simulink model "platforma3"  (Simulink 7.9)
settings: Solver=ode23  StartTime=0.0  StopTime=60  RelTol=1e-8
values from neighbouring files (symbols this model uses):
  a = 0.365    [REX.m]
  b = 0.365    [REX.m]
  c = 0.387    [REX.m]
  d = 0.387    [REX.m]
  enk = 0    [REX.m]
  eta_G = 0.72    [przekladnia_203126.m]    (also in przekladnia_203128.m = 0.64; przekladnia_223095.m = 0.75)
  fr = 0.1    [REX.m]
  g = 9.81    [REX.m]
  i = 113    [przekladnia_203126.m]    (also in przekladnia_203128.m = 150; przekladnia_223095.m)
  I_0 = 0.834    [silnik_136211.m]    (also in silnik_305014.m = 0.485)
  Ik = 0.15    [REX.m]
  Ip = I    (= 4.4)    [REX.m]
  J_R = 209*10^(-3)*(10^(-2))^2    (= 2.09e-05)    [silnik_136211.m]    (also in silnik_305014.m = 3.3e-06)
  JC = 0.15*10^-3    (= 0.00015)    [przekladnia_203126.m]    (also in przekladnia_203128.m; przekladnia_223095.m)
  k1 = 1    [REX.m]
  k2 = 1    [REX.m]
  k_M = 32.8 *10^(-3)    (= 0.0328)    [silnik_136211.m]    (also in silnik_305014.m = 0.0205)
  Kd = 300    [REX.m]
  mi = 0.9    [REX.m]
  mp = 45    [REX.m]
  n_0 = 9730    [silnik_136211.m]    (also in silnik_305014.m = 16700)
  n_n = 10400    [silnik_136211.m]    (also in silnik_305014.m = 16200)
  omega = 0.15    [REX.m]
  R = 10    [REX.m]
  r = 0.127    [REX.m]
  tt = 0.387    [REX.m]
  vd = 1.5    [REX.m]
undefined symbols (not defined in the file or in its folder): dm, F, f0, f1, Irstop, sigB, sigG, sigR, v0
settings Model: Creator=mat  LastModifiedBy=student
settings DebuggingCC: FcnCallInpInsideContextMsg=Use local settings
settings GRTTargetCC: CombineOutputUpdateFcns=off  GRTInterface=on

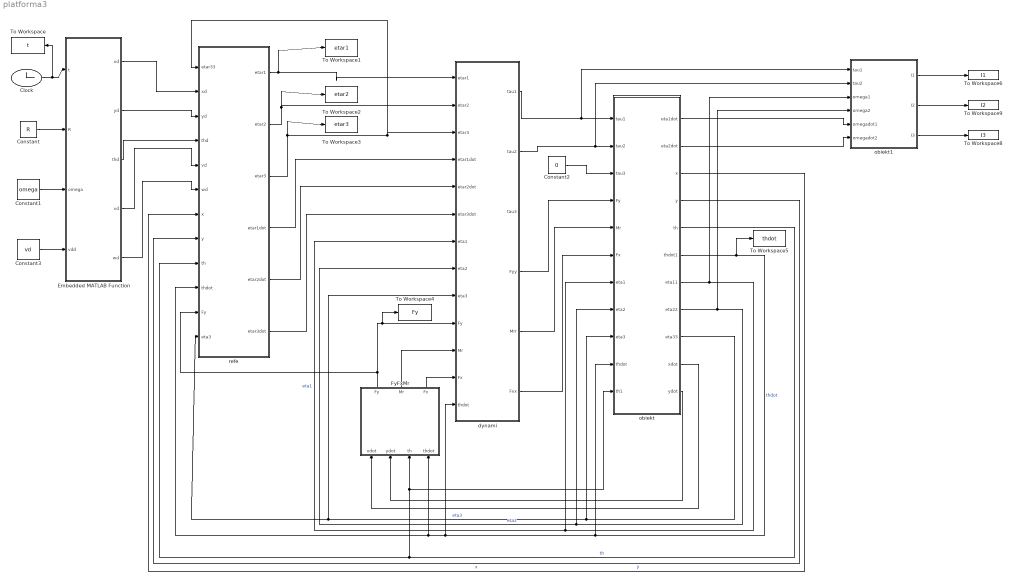
== system platforma3 ==
  Clock : Clock
  Constant : Constant  Value=R
  Constant1 : Constant  Value=omega
  Constant2 : Constant  Value=0
  Constant3 : Constant  Value=vd
  Embedded MATLAB Function : MATLAB Function  TreatAsAtomicUnit=on
  FyFxMr : Subsystem
  To Workspace : ToWorkspace  VariableName=t  SampleTime=-1
  To Workspace1 : ToWorkspace  VariableName=etar1  SampleTime=-1
  To Workspace2 : ToWorkspace  VariableName=etar2  SampleTime=-1
  To Workspace3 : ToWorkspace  VariableName=etar3  SampleTime=-1
  To Workspace4 : ToWorkspace  VariableName=Fy  SampleTime=-1
  To Workspace5 : ToWorkspace  VariableName=thdot  SampleTime=-1
  To Workspace6 : ToWorkspace  VariableName=I1  SampleTime=-1
  To Workspace8 : ToWorkspace  VariableName=I3  SampleTime=-1
  To Workspace9 : ToWorkspace  VariableName=I2  SampleTime=-1
  dynami : Subsystem
  obiekt : Subsystem
  obiekt1 : Subsystem
  refe : Subsystem
  wires:
  Clock/1 -> Embedded MATLAB Function/1(t), To Workspace/1
  Constant/1 -> Embedded MATLAB Function/2(R)
  Constant1/1 -> Embedded MATLAB Function/3(omega)
  dynami/1(tau1) -> obiekt/1(tau1), obiekt1/1(tau1)
  dynami/2(tau2) -> obiekt/2(tau2), obiekt1/2(tau2)
  FyFxMr/3(Fx) -> dynami/12(Fx)
  dynami/4(Fyy) -> obiekt/4(Fy)
  dynami/5(Mrr) -> obiekt/5(Mr)
  dynami/6(Fxx) -> obiekt/6(Fx)
  obiekt/9(eta33) -> obiekt/9(eta3), dynami/9(eta3), refe/12(eta3)  "eta3"
  obiekt/8(eta22) -> obiekt1/4(omega2), obiekt/8(eta2), dynami/8(eta2)  "eta2"
  obiekt/7(eta11) -> obiekt1/3(omega1), obiekt/7(eta1), dynami/7(eta1)  "eta1"
  Embedded MATLAB Function/1(xd) -> refe/2(xd)
  Embedded MATLAB Function/2(yd) -> refe/3(yd)
  Embedded MATLAB Function/4(vd) -> refe/5(vd)
  Embedded MATLAB Function/5(wd) -> refe/6(wd)
  refe/1(etar1) -> dynami/1(etar1), To Workspace1/1
  refe/2(etar2) -> dynami/2(etar2), To Workspace2/1
  refe/3(etar3) -> dynami/3(etar3), refe/1(etar33), To Workspace3/1
  refe/4(etar1dot) -> dynami/4(etar1dot)
  refe/5(etar2dot) -> dynami/5(etar2dot)
  refe/6(etar3dot) -> dynami/6(etar3dot)
  FyFxMr/2(Mr) -> dynami/11(Mr)
  FyFxMr/1(Fy) -> refe/11(Fy), dynami/10(Fy), To Workspace4/1
  obiekt/3(x) -> refe/7(x)  "x"
  obiekt/4(y) -> refe/8(y)  "y"
  obiekt/5(th) -> refe/9(th), FyFxMr/3(th), obiekt/11(th1)  "th"
  obiekt/6(thdot1) -> dynami/13(thdot), FyFxMr/4(thdot), refe/10(thdot), obiekt/10(thdot), To Workspace5/1  "thdot"
  obiekt/11(ydot) -> FyFxMr/2(ydot)
  obiekt/10(xdot) -> FyFxMr/1(xdot)
  Embedded MATLAB Function/3(thd) -> refe/4(thd)
  Constant2/1 -> obiekt/3(tau3)
  obiekt/2(eta2dot) -> obiekt1/6(omegadot2)
  obiekt/1(eta1dot) -> obiekt1/5(omegadot1)
  Constant3/1 -> Embedded MATLAB Function/4(vdd)
  obiekt1/1(I1) -> To Workspace6/1
  obiekt1/2(I2) -> To Workspace9/1
  obiekt1/3(I3) -> To Workspace8/1

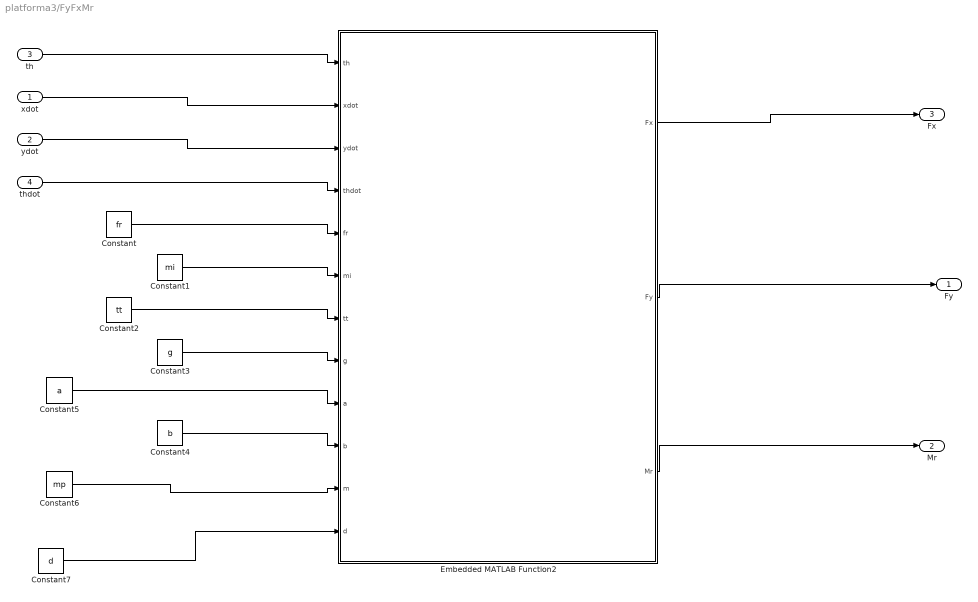
== system platforma3/FyFxMr ==
  xdot : Inport
  ydot : Inport  Port=2
  th : Inport  Port=3
  thdot : Inport  Port=4
  Constant : Constant  Value=fr
  Constant1 : Constant  Value=mi
  Constant2 : Constant  Value=tt
  Constant3 : Constant  Value=g
  Constant4 : Constant  Value=b
  Constant5 : Constant  Value=a
  Constant6 : Constant  Value=mp
  Constant7 : Constant  Value=d
  Embedded MATLAB Function2 : MATLAB Function  TreatAsAtomicUnit=on
  Fy : Outport
  Mr : Outport  Port=2
  Fx : Outport  Port=3
  wires:
  th/1 -> Embedded MATLAB Function2/1(th)
  thdot/1 -> Embedded MATLAB Function2/4(thdot)
  Constant/1 -> Embedded MATLAB Function2/5(fr)
  Constant1/1 -> Embedded MATLAB Function2/6(mi)
  Constant2/1 -> Embedded MATLAB Function2/7(tt)
  Constant3/1 -> Embedded MATLAB Function2/8(g)
  Constant5/1 -> Embedded MATLAB Function2/9(a)
  Constant4/1 -> Embedded MATLAB Function2/10(b)
  Constant6/1 -> Embedded MATLAB Function2/11(m)
  Constant7/1 -> Embedded MATLAB Function2/12(d)
  Embedded MATLAB Function2/3(Mr) -> Mr/1
  Embedded MATLAB Function2/2(Fy) -> Fy/1
  Embedded MATLAB Function2/1(Fx) -> Fx/1
  xdot/1 -> Embedded MATLAB Function2/2(xdot)
  ydot/1 -> Embedded MATLAB Function2/3(ydot)

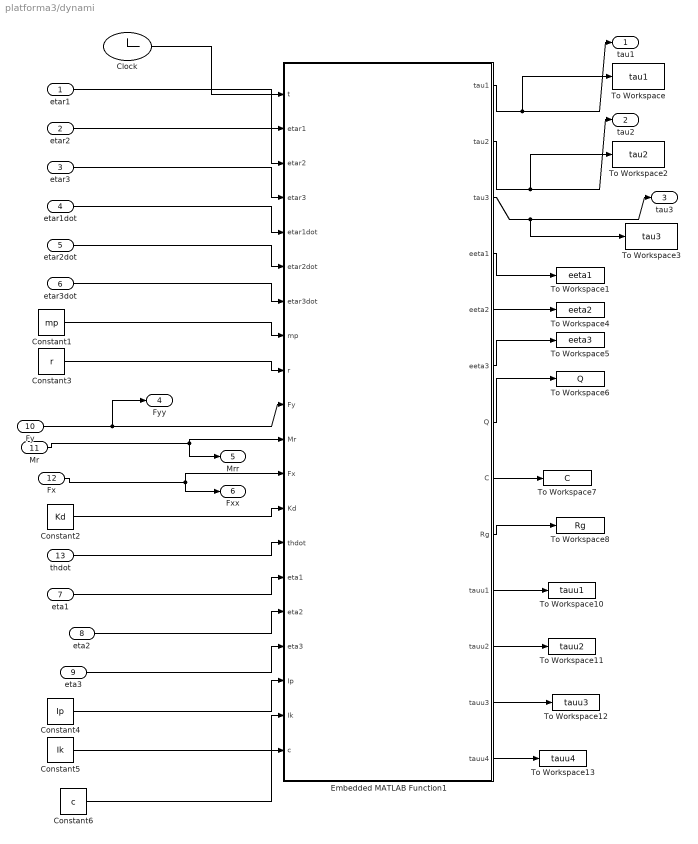
== system platforma3/dynami ==
  etar1 : Inport
  etar2 : Inport  Port=2
  etar3 : Inport  Port=3
  etar1dot : Inport  Port=4
  etar2dot : Inport  Port=5
  etar3dot : Inport  Port=6
  eta1 : Inport  Port=7
  eta2 : Inport  Port=8
  eta3 : Inport  Port=9
  Fy : Inport  Port=10
  Mr : Inport  Port=11
  Fx : Inport  Port=12
  thdot : Inport  Port=13
  Clock : Clock
  Constant1 : Constant  Value=mp
  Constant2 : Constant  Value=Kd
  Constant3 : Constant  Value=r
  Constant4 : Constant  Value=Ip
  Constant5 : Constant  Value=Ik
  Constant6 : Constant  Value=c
  Embedded MATLAB Function1 : MATLAB Function  TreatAsAtomicUnit=on
  To Workspace : ToWorkspace  VariableName=tau1  SampleTime=-1
  To Workspace1 : ToWorkspace  VariableName=eeta1  SampleTime=-1
  To Workspace10 : ToWorkspace  VariableName=tauu1  SampleTime=-1
  To Workspace11 : ToWorkspace  VariableName=tauu2  SampleTime=-1
  To Workspace12 : ToWorkspace  VariableName=tauu3  SampleTime=-1
  To Workspace13 : ToWorkspace  VariableName=tauu4  SampleTime=-1
  To Workspace2 : ToWorkspace  VariableName=tau2  SampleTime=-1
  To Workspace3 : ToWorkspace  VariableName=tau3  SampleTime=-1
  To Workspace4 : ToWorkspace  VariableName=eeta2  SampleTime=-1
  To Workspace5 : ToWorkspace  VariableName=eeta3  SampleTime=-1
  To Workspace6 : ToWorkspace  VariableName=Q  SampleTime=-1
  To Workspace7 : ToWorkspace  VariableName=C  SampleTime=-1
  To Workspace8 : ToWorkspace  VariableName=Rg  SampleTime=-1
  tau1 : Outport
  tau2 : Outport  Port=2
  tau3 : Outport  Port=3
  Fyy : Outport  Port=4
  Mrr : Outport  Port=5
  Fxx : Outport  Port=6
  wires:
  etar1/1 -> Embedded MATLAB Function1/2(etar1)
  etar2/1 -> Embedded MATLAB Function1/3(etar2)
  Embedded MATLAB Function1/1(tau1) -> tau1/1, To Workspace/1
  Embedded MATLAB Function1/2(tau2) -> tau2/1, To Workspace2/1
  Fy/1 -> Fyy/1, Embedded MATLAB Function1/10(Fy)
  Mr/1 -> Mrr/1, Embedded MATLAB Function1/11(Mr)
  Fx/1 -> Fxx/1, Embedded MATLAB Function1/12(Fx)
  Embedded MATLAB Function1/6(eeta3) -> To Workspace5/1
  Embedded MATLAB Function1/3(tau3) -> tau3/1, To Workspace3/1
  Embedded MATLAB Function1/4(eeta1) -> To Workspace1/1
  Embedded MATLAB Function1/5(eeta2) -> To Workspace4/1
  Embedded MATLAB Function1/7(Q) -> To Workspace6/1
  Embedded MATLAB Function1/8(C) -> To Workspace7/1
  Embedded MATLAB Function1/9(Rg) -> To Workspace8/1
  Constant5/1 -> Embedded MATLAB Function1/19(Ik)
  Constant4/1 -> Embedded MATLAB Function1/18(Ip)
  eta3/1 -> Embedded MATLAB Function1/17(eta3)
  eta2/1 -> Embedded MATLAB Function1/16(eta2)
  eta1/1 -> Embedded MATLAB Function1/15(eta1)
  thdot/1 -> Embedded MATLAB Function1/14(thdot)
  Constant2/1 -> Embedded MATLAB Function1/13(Kd)
  Constant3/1 -> Embedded MATLAB Function1/9(r)
  Constant1/1 -> Embedded MATLAB Function1/8(mp)
  etar3dot/1 -> Embedded MATLAB Function1/7(etar3dot)
  etar2dot/1 -> Embedded MATLAB Function1/6(etar2dot)
  etar1dot/1 -> Embedded MATLAB Function1/5(etar1dot)
  etar3/1 -> Embedded MATLAB Function1/4(etar3)
  Embedded MATLAB Function1/13(tauu4) -> To Workspace13/1
  Embedded MATLAB Function1/12(tauu3) -> To Workspace12/1
  Embedded MATLAB Function1/11(tauu2) -> To Workspace11/1
  Embedded MATLAB Function1/10(tauu1) -> To Workspace10/1
  Clock/1 -> Embedded MATLAB Function1/1(t)
  Constant6/1 -> Embedded MATLAB Function1/20(c)

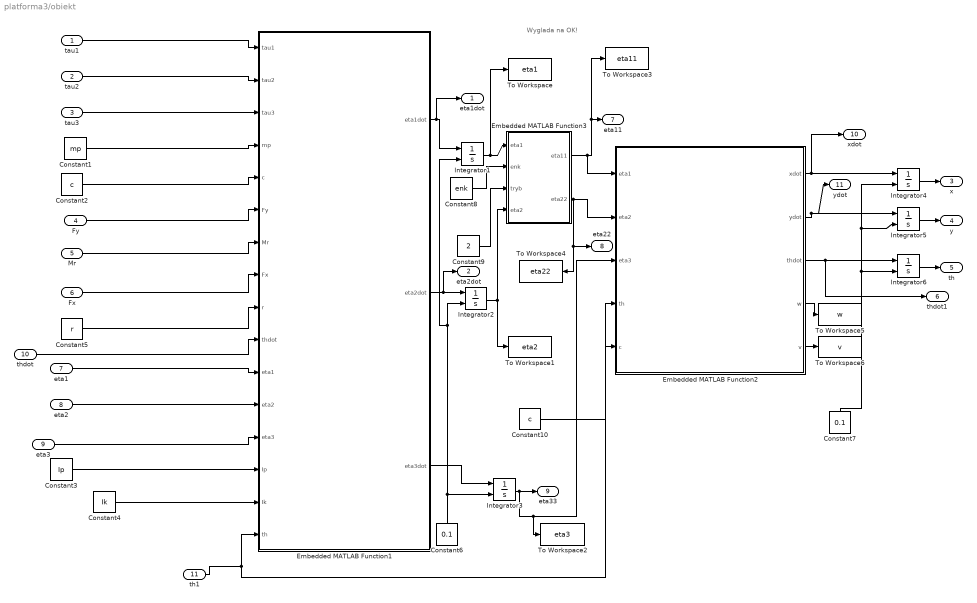
== system platforma3/obiekt ==
  note: Wyglada na OK!
  tau1 : Inport
  tau2 : Inport  Port=2
  tau3 : Inport  Port=3
  Fy : Inport  Port=4
  Mr : Inport  Port=5
  Fx : Inport  Port=6
  eta1 : Inport  Port=7
  eta2 : Inport  Port=8
  eta3 : Inport  Port=9
  thdot : Inport  Port=10
  th1 : Inport  Port=11
  Constant1 : Constant  Value=mp
  Constant10 : Constant  Value=c
  Constant2 : Constant  Value=c
  Constant3 : Constant  Value=Ip
  Constant4 : Constant  Value=Ik
  Constant5 : Constant  Value=r
  Constant6 : Constant  Value=0.1
  Constant7 : Constant  Value=0.1
  Constant8 : Constant  Value=enk
  Constant9 : Constant  Value=2
  Embedded MATLAB Function1 : MATLAB Function  TreatAsAtomicUnit=on
  Embedded MATLAB Function2 : MATLAB Function  TreatAsAtomicUnit=on
  Embedded MATLAB Function3 : MATLAB Function  TreatAsAtomicUnit=on
  Integrator{1..6} (6 alike) : Integrator  InitialConditionSource=external
  To Workspace : ToWorkspace  VariableName=eta1  SampleTime=-1
  To Workspace1 : ToWorkspace  VariableName=eta2  SampleTime=-1
  To Workspace2 : ToWorkspace  VariableName=eta3  SampleTime=-1
  To Workspace3 : ToWorkspace  VariableName=eta11  SampleTime=-1
  To Workspace4 : ToWorkspace  VariableName=eta22  SampleTime=-1
  To Workspace5 : ToWorkspace  VariableName=w  SampleTime=-1
  To Workspace6 : ToWorkspace  VariableName=v  SampleTime=-1
  eta1dot : Outport
  eta2dot : Outport  Port=2
  x : Outport  Port=3
  y : Outport  Port=4
  th : Outport  Port=5
  thdot1 : Outport  Port=6
  eta11 : Outport  Port=7
  eta22 : Outport  Port=8
  eta33 : Outport  Port=9
  xdot : Outport  Port=10
  ydot : Outport  Port=11
  wires:
  Constant1/1 -> Embedded MATLAB Function1/4(mp)
  Fy/1 -> Embedded MATLAB Function1/6(Fy)
  Mr/1 -> Embedded MATLAB Function1/7(Mr)
  tau1/1 -> Embedded MATLAB Function1/1(tau1)
  tau3/1 -> Embedded MATLAB Function1/3(tau3)
  tau2/1 -> Embedded MATLAB Function1/2(tau2)
  eta3/1 -> Embedded MATLAB Function1/13(eta3)
  eta1/1 -> Embedded MATLAB Function1/11(eta1)
  eta2/1 -> Embedded MATLAB Function1/12(eta2)
  thdot/1 -> Embedded MATLAB Function1/10(thdot)
  Fx/1 -> Embedded MATLAB Function1/8(Fx)
  Constant5/1 -> Embedded MATLAB Function1/9(r)
  Embedded MATLAB Function1/3(eta3dot) -> Integrator3/1
  Embedded MATLAB Function1/2(eta2dot) -> Integrator2/1, eta2dot/1
  Embedded MATLAB Function1/1(eta1dot) -> Integrator1/1, eta1dot/1
  Constant2/1 -> Embedded MATLAB Function1/5(c)
  Constant3/1 -> Embedded MATLAB Function1/14(Ip)
  Constant4/1 -> Embedded MATLAB Function1/15(Ik)
  Constant6/1 -> Integrator1/2, Integrator2/2, Integrator3/2
  Integrator3/1 -> eta33/1, Embedded MATLAB Function2/3(eta3), To Workspace2/1
  Embedded MATLAB Function2/1(xdot) -> Integrator4/1, xdot/1
  Integrator4/1 -> x/1
  Integrator5/1 -> y/1
  Embedded MATLAB Function2/2(ydot) -> Integrator5/1, ydot/1
  Integrator6/1 -> th/1
  Constant7/1 -> Integrator4/2, Integrator5/2, Integrator6/2
  Embedded MATLAB Function2/3(thdot) -> Integrator6/1, thdot1/1
  th1/1 -> Embedded MATLAB Function1/16(th), Embedded MATLAB Function2/4(th)
  Integrator1/1 -> Embedded MATLAB Function3/1(eta1), To Workspace/1
  Embedded MATLAB Function3/1(eta11) -> Embedded MATLAB Function2/1(eta1), To Workspace3/1, eta11/1
  Integrator2/1 -> Embedded MATLAB Function3/4(eta2), To Workspace1/1
  Embedded MATLAB Function3/2(eta22) -> Embedded MATLAB Function2/2(eta2), eta22/1, To Workspace4/1
  Constant8/1 -> Embedded MATLAB Function3/2(enk)
  Constant9/1 -> Embedded MATLAB Function3/3(tryb)
  Constant10/1 -> Embedded MATLAB Function2/5(c)
  Embedded MATLAB Function2/4(w) -> To Workspace5/1
  Embedded MATLAB Function2/5(v) -> To Workspace6/1

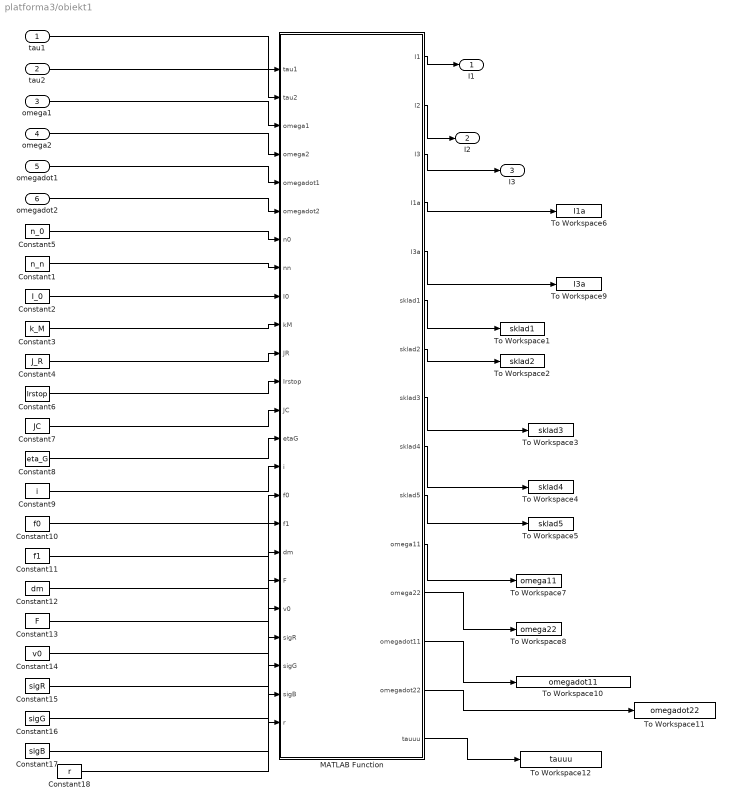
== system platforma3/obiekt1 ==
  tau1 : Inport
  tau2 : Inport  Port=2
  omega1 : Inport  Port=3
  omega2 : Inport  Port=4
  omegadot1 : Inport  Port=5
  omegadot2 : Inport  Port=6
  Constant1 : Constant  Value=n_n
  Constant10 : Constant  Value=f0
  Constant11 : Constant  Value=f1
  Constant12 : Constant  Value=dm
  Constant13 : Constant  Value=F
  Constant14 : Constant  Value=v0
  Constant15 : Constant  Value=sigR
  Constant16 : Constant  Value=sigG
  Constant17 : Constant  Value=sigB
  Constant18 : Constant  Value=r
  Constant2 : Constant  Value=I_0
  Constant3 : Constant  Value=k_M
  Constant4 : Constant  Value=J_R
  Constant5 : Constant  Value=n_0
  Constant6 : Constant  Value=Irstop
  Constant7 : Constant  Value=JC
  Constant8 : Constant  Value=eta_G
  Constant9 : Constant  Value=i
  MATLAB Function : MATLAB Function  TreatAsAtomicUnit=on
  To Workspace1 : ToWorkspace  VariableName=sklad1  SampleTime=-1
  To Workspace10 : ToWorkspace  VariableName=omegadot11  SampleTime=-1
  To Workspace11 : ToWorkspace  VariableName=omegadot22  SampleTime=-1
  To Workspace12 : ToWorkspace  VariableName=tauuu  SampleTime=-1
  To Workspace2 : ToWorkspace  VariableName=sklad2  SampleTime=-1
  To Workspace3 : ToWorkspace  VariableName=sklad3  SampleTime=-1
  To Workspace4 : ToWorkspace  VariableName=sklad4  SampleTime=-1
  To Workspace5 : ToWorkspace  VariableName=sklad5  SampleTime=-1
  To Workspace6 : ToWorkspace  VariableName=I1a  SampleTime=-1
  To Workspace7 : ToWorkspace  VariableName=omega11  SampleTime=-1
  To Workspace8 : ToWorkspace  VariableName=omega22  SampleTime=-1
  To Workspace9 : ToWorkspace  VariableName=I3a  SampleTime=-1
  I1 : Outport
  I2 : Outport  Port=2
  I3 : Outport  Port=3
  wires:
  tau1/1 -> MATLAB Function/1(tau1)
  tau2/1 -> MATLAB Function/2(tau2)
  omega1/1 -> MATLAB Function/3(omega1)
  omega2/1 -> MATLAB Function/4(omega2)
  omegadot1/1 -> MATLAB Function/5(omegadot1)
  omegadot2/1 -> MATLAB Function/6(omegadot2)
  MATLAB Function/1(I1) -> I1/1
  MATLAB Function/2(I2) -> I2/1
  MATLAB Function/3(I3) -> I3/1
  Constant5/1 -> MATLAB Function/7(n0)
  Constant1/1 -> MATLAB Function/8(nn)
  Constant2/1 -> MATLAB Function/9(I0)
  Constant3/1 -> MATLAB Function/10(kM)
  Constant4/1 -> MATLAB Function/11(JR)
  Constant6/1 -> MATLAB Function/12(Irstop)
  Constant7/1 -> MATLAB Function/13(JC)
  Constant8/1 -> MATLAB Function/14(etaG)
  Constant9/1 -> MATLAB Function/15(i)
  Constant10/1 -> MATLAB Function/16(f0)
  Constant11/1 -> MATLAB Function/17(f1)
  Constant12/1 -> MATLAB Function/18(dm)
  Constant13/1 -> MATLAB Function/19(F)
  Constant14/1 -> MATLAB Function/20(v0)
  Constant15/1 -> MATLAB Function/21(sigR)
  Constant16/1 -> MATLAB Function/22(sigG)
  Constant17/1 -> MATLAB Function/23(sigB)
  MATLAB Function/4(I1a) -> To Workspace6/1
  MATLAB Function/5(I3a) -> To Workspace9/1
  MATLAB Function/10(sklad5) -> To Workspace5/1
  MATLAB Function/9(sklad4) -> To Workspace4/1
  MATLAB Function/8(sklad3) -> To Workspace3/1
  MATLAB Function/7(sklad2) -> To Workspace2/1
  MATLAB Function/6(sklad1) -> To Workspace1/1
  Constant18/1 -> MATLAB Function/24(r)
  MATLAB Function/11(omega11) -> To Workspace7/1
  MATLAB Function/12(omega22) -> To Workspace8/1
  MATLAB Function/13(omegadot11) -> To Workspace10/1
  MATLAB Function/14(omegadot22) -> To Workspace11/1
  MATLAB Function/15(tauuu) -> To Workspace12/1

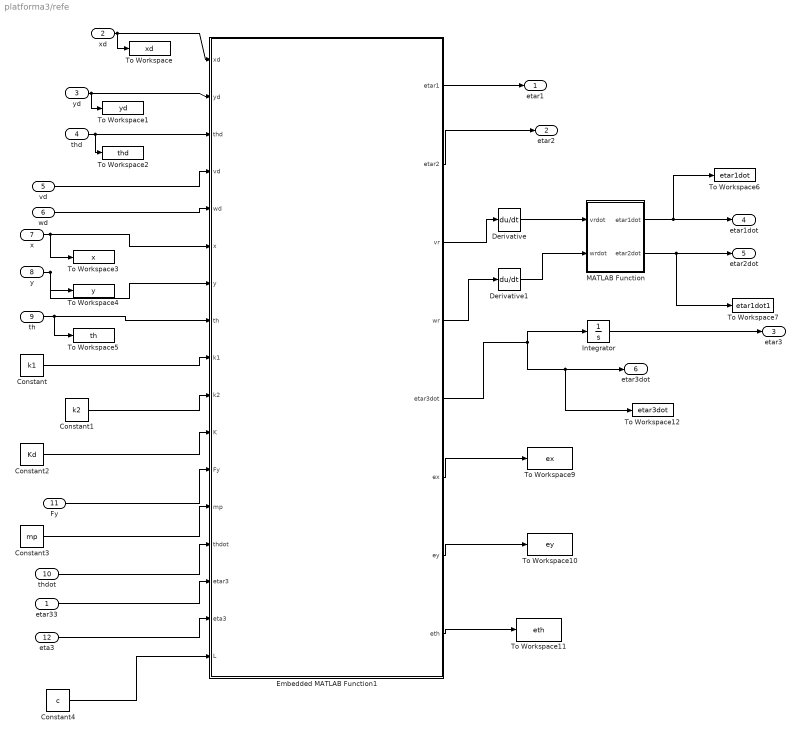
== system platforma3/refe ==
  etar33 : Inport
  xd : Inport  Port=2
  yd : Inport  Port=3
  thd : Inport  Port=4
  vd : Inport  Port=5
  wd : Inport  Port=6
  x : Inport  Port=7
  y : Inport  Port=8
  th : Inport  Port=9
  thdot : Inport  Port=10
  Fy : Inport  Port=11
  eta3 : Inport  Port=12
  Constant : Constant  Value=k1
  Constant1 : Constant  Value=k2
  Constant2 : Constant  Value=Kd
  Constant3 : Constant  Value=mp
  Constant4 : Constant  Value=c
  Derivative : Derivative
  Derivative1 : Derivative
  Embedded MATLAB Function1 : MATLAB Function  TreatAsAtomicUnit=on
  Integrator : Integrator  InitialCondition=0.1
  MATLAB Function : MATLAB Function  TreatAsAtomicUnit=on
  To Workspace : ToWorkspace  VariableName=xd  SampleTime=-1
  To Workspace1 : ToWorkspace  VariableName=yd  SampleTime=-1
  To Workspace10 : ToWorkspace  VariableName=ey  SampleTime=-1
  To Workspace11 : ToWorkspace  VariableName=eth  SampleTime=-1
  To Workspace12 : ToWorkspace  VariableName=etar3dot  SampleTime=-1
  To Workspace2 : ToWorkspace  VariableName=thd  SampleTime=-1
  To Workspace3 : ToWorkspace  VariableName=x  SampleTime=-1
  To Workspace4 : ToWorkspace  VariableName=y  SampleTime=-1
  To Workspace5 : ToWorkspace  VariableName=th  SampleTime=-1
  To Workspace6 : ToWorkspace  VariableName=etar1dot  SampleTime=-1
  To Workspace7 : ToWorkspace  VariableName=etar1dot1  SampleTime=-1
  To Workspace9 : ToWorkspace  VariableName=ex  SampleTime=-1
  etar1 : Outport
  etar2 : Outport  Port=2
  etar3 : Outport  Port=3
  etar1dot : Outport  Port=4
  etar2dot : Outport  Port=5
  etar3dot : Outport  Port=6
  wires:
  xd/1 -> Embedded MATLAB Function1/1(xd), To Workspace/1
  yd/1 -> Embedded MATLAB Function1/2(yd), To Workspace1/1
  thd/1 -> Embedded MATLAB Function1/3(thd), To Workspace2/1
  vd/1 -> Embedded MATLAB Function1/4(vd)
  wd/1 -> Embedded MATLAB Function1/5(wd)
  x/1 -> Embedded MATLAB Function1/6(x), To Workspace3/1
  y/1 -> Embedded MATLAB Function1/7(y), To Workspace4/1
  th/1 -> Embedded MATLAB Function1/8(th), To Workspace5/1
  Constant/1 -> Embedded MATLAB Function1/9(k1)
  Constant1/1 -> Embedded MATLAB Function1/10(k2)
  Embedded MATLAB Function1/1(etar1) -> etar1/1
  Embedded MATLAB Function1/2(etar2) -> etar2/1
  Integrator/1 -> etar3/1
  etar33/1 -> Embedded MATLAB Function1/15(etar3)
  Constant2/1 -> Embedded MATLAB Function1/11(K)
  Fy/1 -> Embedded MATLAB Function1/12(Fy)
  Constant3/1 -> Embedded MATLAB Function1/13(mp)
  thdot/1 -> Embedded MATLAB Function1/14(thdot)
  eta3/1 -> Embedded MATLAB Function1/16(eta3)
  Embedded MATLAB Function1/5(etar3dot) -> Integrator/1, etar3dot/1, To Workspace12/1
  Embedded MATLAB Function1/3(vr) -> Derivative/1
  Embedded MATLAB Function1/4(wr) -> Derivative1/1
  Derivative/1 -> MATLAB Function/1(vrdot)
  Derivative1/1 -> MATLAB Function/2(wrdot)
  MATLAB Function/1(etar1dot) -> etar1dot/1, To Workspace6/1
  MATLAB Function/2(etar2dot) -> etar2dot/1, To Workspace7/1
  Embedded MATLAB Function1/6(ex) -> To Workspace9/1
  Embedded MATLAB Function1/7(ey) -> To Workspace10/1
  Embedded MATLAB Function1/8(eth) -> To Workspace11/1
  Constant4/1 -> Embedded MATLAB Function1/17(L)

== matlab function dynami/Embedded MATLAB Function1 ==
  data: t input double; etar1 input double; etar2 input double; tau1 output double; tau2 output double; tau3 output double; eeta1 output double; eeta2 output double; eeta3 output double; Q output double; C output double; Rg output double; etar3 input double; etar1dot input double; etar2dot input double; etar3dot input double; mp input double; r input double; Fy input double; Mr input double; Fx input double; Kd input double; thdot input double; eta1 input double; eta2 input double; eta3 input double; Ip input double; Ik input double; tauu1 output double; tauu2 output double; tauu3 output double; tauu4 output double; c input double
function [tau1,tau2,tau3, eeta1,eeta2,eeta3, Q, C, Rg,...
    tauu1, tauu2, tauu3, tauu4]  =fcn(t,etar1, etar2,...
etar3, etar1dot, etar2dot, etar3dot, mp,r, Fy,Mr, Fx,Kd, thdot,...
eta1,eta2,eta3,Ip, Ik, c)

%c=0.31;
tau=zeros(3,1);

eeta1=eta1-etar1;
eeta2=eta2-etar2;
eeta3=eta3-etar3;

invB =[r/2 0 0;
       0 r/2 0;
       0 0 1];
   
Q=[mp+Ip/c^2+4*Ik/r^2 mp-1/c^2*Ip 0;
   mp-1/c^2*Ip mp+Ip/c^2+4*Ik/r^2 0;
   0 0 mp];

C=[0 0 -mp*thdot;
   0 0 -mp*thdot;
   mp*thdot mp*thdot 0];
  

Rg=[-Fx-Mr/c;-Fx+Mr/c;-Fy];
tauu1=invB*Q*[etar1dot;etar2dot;etar3dot];
tauu2=invB*C*[etar1;etar2;etar3];
tauu3=invB*Rg;
tauu4=invB*Kd*[eeta1;eeta2;eeta3];

% tau=invB*(Q*[etar1dot;etar2dot;etar3dot]+C*[etar1;etar2;etar3]+Rg-Kd*[eeta1;eeta2;eeta3]);
tau=tauu1+tauu2+tauu3-tauu4;

tau1=tau(1,1);
tau2=tau(2,1);
tau3=tau(3,1);

if tau1>50
    tau1=70;
elseif tau1<-70
    tau1=-70;
end;

if tau2>70
    tau2=70;
elseif tau2<-70
    tau2=-70;
end;

== matlab function Embedded MATLAB Function ==
  data: xd output double; yd output double; thd output double; vd output double; wd output double; t input double; R input double; omega input double; vdd input double
 function [ xd, yd, thd,  vd, wd] = generator(t, R, omega, vdd)
% This block supports the Embedded MATLAB subset.
% See the help menu for details. 

% L=0.315;

% if t<20
xd=R*sin(omega*t);
yd=-R*cos(omega*t);
thd=omega*t;
% else
% xd=R*sin(omega*20)+1*(t-20);
% yd=-R*cos(omega*20);
% thd=omega*20;
    
% end;


% thd=pi/4;
% xd=t;
% yd=t;

 vd=vdd;
 wd=omega;

== matlab function obiekt/Embedded MATLAB Function1 ==
  data: tau1 input double; tau2 input double; tau3 input double; mp input double; c input double; Fy input double; Mr input double; Fx input double; r input double; thdot input double; eta1 input double; eta1dot output double; eta2dot output double; eta3dot output double; eta2 input double; eta3 input double; Ip input double; Ik input double; th input double
function [eta1dot,eta2dot,eta3dot]    =fcn(tau1, tau2, tau3, mp, c, Fy, Mr, Fx, r, thdot,...
    eta1,eta2,eta3, Ip, Ik, th)
%c=0.31;
etadot=zeros(3,1);
qdot=zeros(3,1);

B =[2/r 0 0;
    0 2/r 0;
    0 0 1];

Q=[mp+Ip/c^2+4*Ik/r^2 mp-1/c^2*Ip 0;
   mp-1/c^2*Ip mp+Ip/c^2+4*Ik/r^2 0;
   0 0 mp];

C=[0 0 -mp*thdot;
   0 0 -mp*thdot;
   mp*thdot mp*thdot 0];
    
Rg=[-Fx-Mr/c;-Fx+Mr/c;-Fy];

detQ=det(Q);
% etadot=inv(Q)*(B*[tau1;tau2;tau3]-C*[eta1;eta2;eta3]-Rg);
etadot=inv(Q)*(B*[tau1;tau2;tau3]-C*[eta1;eta2;eta3]-Rg);

eta1dot=etadot(1,1);
eta2dot=etadot(2,1);
eta3dot=etadot(3,1);

== matlab function FyFxMr/Embedded MATLAB Function2 ==
  data: th input double; xdot input double; ydot input double; Fx output double; thdot input double; fr input double; mi input double; tt input double; g input double; Fy output double; Mr output double; a input double; b input double; m input double; d input double
function [Fx, Fy, Mr] = fcn(th, xdot, ydot, thdot, fr, mi, tt, g,a,b, m, d)
%#eml

R=[cos(th) -sin(th);
    sin(th) cos(th)];

xx=inv(R)*[xdot; ydot];
% xx=[xdot; ydot];

x1p=xx(1,1)-tt*thdot;
x2p=xx(1,1)+tt*thdot;

y1p=xx(2,1)+a*thdot;
y3p=xx(2,1)-b*thdot;

Fx=fr*m*g*(sign(x1p)+sign(x2p))/2;
Fy=mi*m*g*(b*sign(y1p)+a*sign(y3p))/(a+b);
Mr=mi*a*b*m*g*(sign(y1p)-sign(y3p))/(a+b) + fr*tt*m*g*(sign(x2p)-sign(x1p))/2;

== matlab function refe/MATLAB Function ==
  data: vrdot input double; etar1dot output double; wrdot input double; etar2dot output double
function [etar1dot, etar2dot] = fcn(vrdot, wrdot)
%#codegen
L=0.31;
etar1dot=(vrdot-L*wrdot)/2;
etar2dot=(vrdot+L*wrdot)/2;

== matlab function refe/Embedded MATLAB Function1 ==
  data: xd input double; yd input double; thd input double; vd input double; wd input double; x input double; y input double; th input double; k1 input double; etar1 output double; etar2 output double; vr output double; wr output double; k2 input double; etar3dot output double; K input double; Fy input double; mp input double; thdot input double; etar3 input double; eta3 input double; ex output double; ey output double; eth output double; L input double
    function [etar1,etar2, vr, wr, etar3dot, ex,ey,eth] =fcn(xd,yd,thd,vd,wd,x,y,th,k1,k2, K, Fy, mp, thdot, etar3, eta3, L)
%L=0.31;
ex=xd-x;
ey=yd-y;
eth=thd-th;

xe=cos(th)*ex+sin(th)*ey;
ye=-sin(th)*ex+cos(th)*ey;
the=eth;

vr=k1*xe+vd*cos(the);
wr=wd+k2*the+vd*ye*sin(the)/the;%sin(the)/the;1!!!!!!!!!!!!!!!!!!!!!!!!!!!

etar1=(vr-L*wr)/2;
etar2=(vr+L*wr)/2;

eeta3=eta3-etar3;

etar3dot=(K*eeta3+Fy-mp*thdot*(etar1+etar2))/mp;

== matlab function obiekt/Embedded MATLAB Function2 ==
  data: eta1 input double; xdot output double; ydot output double; thdot output double; eta2 input double; eta3 input double; th input double; c input double; w output double; v output double
function [xdot,ydot,thdot, w, v]   =fcn(eta1,eta2,eta3,th, c)
%c=0.31;
L=c;

qdot=zeros(3,1);

G=[cos(th) cos(th);
    sin(th) sin(th);
    -1/c 1/c];

qdot=G*[eta1;eta2];

% G=[cos(th) cos(th) -sin(th);
%     sin(th) sin(th) cos(th);
%     -1/c 1/c 0];
% 
% qdot=G*[eta1;eta2;eta3];

xdot=qdot(1,1);
ydot=qdot(2,1);
thdot=qdot(3,1);

v=(eta1+eta2);
w=(eta1-eta2)/(c); %%%%%%%%%%%%!!!

== matlab function obiekt/Embedded MATLAB Function3 ==
  data: eta1 input double; enk input double; tryb input double; eta11 output double; eta22 output double; eta2 input double
function [eta11,eta22]  =fcn(eta1,enk, tryb, eta2)
eta11=0;
eta22=0;
if (tryb==1)
eta11=eta1;
eta22=eta2+randn*enk;
elseif (tryb ==2)
eta11=eta1+randn*enk;
eta22=eta2+randn*enk;
end

== matlab function obiekt1/MATLAB Function ==
  data: tau1 input double; tau2 input double; omega1 input double; I1 output double; I2 output double; omega2 input double; omegadot1 input double; omegadot2 input double; I3 output double; n0 input double; nn input double; I0 input double; kM input double; JR input double; Irstop input double; JC input double; etaG input double; i input double; f0 input double; f1 input double; dm input double; F input double; v0 input double; sigR input double; sigG input double; sigB input double; I1a output double; I3a output double; sklad1 output double; sklad2 output double; sklad3 output double; sklad4 output double; sklad5 output double; r input double; omega11 output double; omega22 output double; omegadot11 output double; omegadot22 output double; tauuu output double
function [I1, I2, I3, I1a, I3a, sklad1, sklad2, sklad3, sklad4, sklad5,...
    omega11, omega22, omegadot11, omegadot22, tauuu  ] = fcn(tau1,...
    tau2, omega1,omega2, omegadot1, omegadot2,...
    n0, nn, I0, kM, JR, Irstop, JC, etaG, i, f0, f1, dm, F, v0, sigR, sigG, sigB, r)
%#codegen

Fc=kM*Irstop;

omega11=2/r*omega1;
omega22=2/r*omega2;

omegadot11=2/r*omegadot1;
omegadot22=2/r*omegadot2;

sklad1=((etaG*i^2*60/(2*pi)*JR+JC)*omegadot11)/(etaG*i*kM);
sklad2=(etaG*i^2*60/(2*pi)*(kM*I0-Fc)/(n0)*omega11)/(etaG*i*kM);


tauuu=tau1/2;

I1a=(tau1/2-(-(etaG*i^2*60/(2*pi)*JR+JC)*omegadot11-etaG*i^2*60/(2*pi)*(kM*I0-Fc)/(n0)*omega11))/(etaG*i*kM); 

I1=(tau1/2)/(etaG*i*kM)+sklad1+sklad2; %OK

I2=(tau2+(etaG*i^2*60/(2*pi)*JR+JC)*omegadot22+etaG*i^2*60/(2*pi)*(kM*I0-Fc)/(n0)*omega22)/(etaG*i*kM);

I3 = 0;

I3a = 0;

sklad3 = 0;
sklad4 = 0;
sklad5 = 0;
